simulink model "Exercitiul2"  (R2016a)
settings: Solver=VariableStepDiscrete  StartTime=0.0  StopTime=2000  RelTol=1e-3
settings Model: Creator=Cristina  LastModifiedBy=Cristina

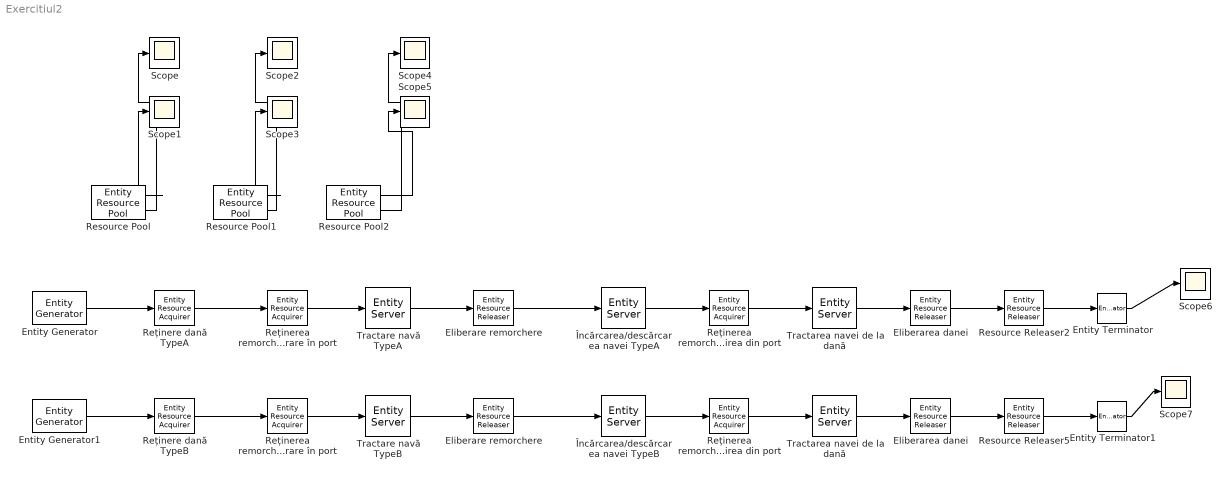
== system Exercitiul2 ==
  Eliberare remorchere : EntityResourceReleaser  InputPortMessageModes=m  OutputPortMessageModes=m  ResourceToRelease=Selected  ResourceName=Remorci
  "Eliberare remorchere " : EntityResourceReleaser  InputPortMessageModes=m  OutputPortMessageModes=m  ResourceToRelease=Selected  ResourceName=Remorci
  Eliberarea danei : EntityResourceReleaser  InputPortMessageModes=m  OutputPortMessageModes=m  ResourceToRelease=Selected  ResourceName=Remorci
  "Eliberarea danei " : EntityResourceReleaser  InputPortMessageModes=m  OutputPortMessageModes=m  ResourceToRelease=Selected  ResourceName=Remorci
  Entity Generator : EntityGenerator  OutputPortMessageModes=m  TimeSource=MATLAB action  IntergenerationTimeAction=dt = 1.7 + rand * 3;  AttributeName=Type  EntityType=Structured  EntityTypeName=TypeA
  Entity Generator1 : EntityGenerator  OutputPortMessageModes=m  TimeSource=MATLAB action  IntergenerationTimeAction=dt = 0.75 + rand * 1.5;  AttributeName=Type  AttributeInitialValue=2  EntityType=Structured  EntityTypeName=TypeB
  Entity Terminator : EntityTerminator  InputPortMessageModes=m  NumberEntitiesArrived=on
      settings: OutputPortMap=o0
  Entity Terminator1 : EntityTerminator  InputPortMessageModes=m  NumberEntitiesArrived=on
      settings: OutputPortMap=o0
  Resource Releaser2 : EntityResourceReleaser  InputPortMessageModes=m  OutputPortMessageModes=m  ResourceToRelease=Selected  ResourceName=DaneA
  Resource Releaser5 : EntityResourceReleaser  InputPortMessageModes=m  OutputPortMessageModes=m  ResourceToRelease=Selected  ResourceName=DaneB
  Resource Pool : EntityResourcePool  ResourceName=DaneA  ResourceAmount=3  AmountInUse=on  AverageUtilization=on
      settings: OutputPortMap=o0,o1
  Resource Pool1 : EntityResourcePool  ResourceName=DaneB  ResourceAmount=2  AmountInUse=on  AverageUtilization=on
      settings: OutputPortMap=o0,o1
  Resource Pool2 : EntityResourcePool  ResourceName=Remorci  ResourceAmount=3  AmountInUse=on  AverageUtilization=on
      settings: OutputPortMap=o0,o1
  Reținere dană TypeA : EntityResourceAcquirer  InputPortMessageModes=m  OutputPortMessageModes=m  NumberWaitingEntities=5  ResourceName=DaneA
      settings: OutputPortMap=o3
  Reținere dană TypeB : EntityResourceAcquirer  InputPortMessageModes=m  OutputPortMessageModes=m  NumberWaitingEntities=5  ResourceName=DaneB
      settings: OutputPortMap=o3
  Reținerea remorcherelor pentru ieșirea din port : EntityResourceAcquirer  InputPortMessageModes=m  OutputPortMessageModes=m  NumberWaitingEntities=5  ResourceName=Remorci  ResourceAmount=2
      settings: OutputPortMap=o3
  "Reținerea remorcherelor pentru ieșirea din port " : EntityResourceAcquirer  InputPortMessageModes=m  OutputPortMessageModes=m  NumberWaitingEntities=5  ResourceName=Remorci
      settings: OutputPortMap=o3
  Reținerea remorcherelor pentru intrare în port : EntityResourceAcquirer  InputPortMessageModes=m  OutputPortMessageModes=m  NumberWaitingEntities=5  ResourceName=Remorci  ResourceAmount=3
      settings: OutputPortMap=o3
  "Reținerea remorcherelor pentru intrare în port " : EntityResourceAcquirer  InputPortMessageModes=m  OutputPortMessageModes=m  NumberWaitingEntities=5  ResourceName=Remorci  ResourceAmount=2
      settings: OutputPortMap=o3
  Scope{,1..7} (8 alike) : Scope
  Tractare navă TypeA : EntityServer  InputPortMessageModes=m  OutputPortMessageModes=m  Capacity=1  ServiceTimeValue=0.5
  Tractare navă TypeB : EntityServer  InputPortMessageModes=m  OutputPortMessageModes=m  Capacity=1  ServiceTimeValue=0.5
  "Tractarea navei de la dană " : EntityServer  InputPortMessageModes=m  OutputPortMessageModes=m  Capacity=1  ServiceTimeValue=0.25  ServiceTimeAction=dt = 6.9 + rand * 3;
  "Tractarea navei de la dană  " : EntityServer  InputPortMessageModes=m  OutputPortMessageModes=m  Capacity=1  ServiceTimeValue=0.25  ServiceTimeAction=dt = 6.9 + rand * 3;
  Încărcarea/descărcarea navei TypeA : EntityServer  InputPortMessageModes=m  OutputPortMessageModes=m  Capacity=1  ServiceTimeSource=MATLAB action  ServiceTimeValue=0.5  ServiceTimeAction=dt = 6.9 + rand * 3;
  Încărcarea/descărcarea navei TypeB : EntityServer  InputPortMessageModes=m  OutputPortMessageModes=m  Capacity=1  ServiceTimeSource=MATLAB action  ServiceTimeValue=0.5  ServiceTimeAction=dt = 1.5 + rand * 1.2;
  wires:
  Entity Generator/1 -> Reținere dană TypeA/1
  Reținere dană TypeA/1 -> Reținerea remorcherelor pentru intrare în port/1
  Reținerea remorcherelor pentru intrare în port/1 -> Tractare navă TypeA/1
  Tractare navă TypeA/1 -> Eliberare remorchere/1
  Eliberare remorchere/1 -> Încărcarea/descărcarea navei TypeA/1
  Încărcarea/descărcarea navei TypeA/1 -> Reținerea remorcherelor pentru ieșirea din port/1
  Reținerea remorcherelor pentru ieșirea din port/1 -> "Tractarea navei de la dană "/1
  "Tractarea navei de la dană "/1 -> Eliberarea danei/1
  Eliberarea danei/1 -> Resource Releaser2/1
  Resource Releaser2/1 -> Entity Terminator/1
  Resource Pool/2 -> Scope/1
  Resource Pool/1 -> Scope1/1
  Resource Pool1/2 -> Scope2/1
  Resource Pool1/1 -> Scope3/1
  Resource Pool2/2 -> Scope4/1
  Resource Pool2/1 -> Scope5/1
  Entity Terminator/1 -> Scope6/1
  Entity Generator1/1 -> Reținere dană TypeB/1
  Reținere dană TypeB/1 -> "Reținerea remorcherelor pentru intrare în port "/1
  Tractare navă TypeB/1 -> "Eliberare remorchere "/1
  "Eliberare remorchere "/1 -> Încărcarea/descărcarea navei TypeB/1
  Încărcarea/descărcarea navei TypeB/1 -> "Reținerea remorcherelor pentru ieșirea din port "/1
  "Reținerea remorcherelor pentru ieșirea din port "/1 -> "Tractarea navei de la dană  "/1
  "Tractarea navei de la dană  "/1 -> "Eliberarea danei "/1
  "Eliberarea danei "/1 -> Resource Releaser5/1
  Resource Releaser5/1 -> Entity Terminator1/1
  "Reținerea remorcherelor pentru intrare în port "/1 -> Tractare navă TypeB/1
  Entity Terminator1/1 -> Scope7/1
